simulink model "testTorchTCP"  (R2023b)
settings: Solver=FixedStepAuto  StartTime=0.0  StopTime=10.0  FixedStep=1  RelTol=1e-3
undefined symbols (not defined in the file or in its folder): inputDataStruct
libraries: instrumentlib x2
settings Model: Creator=pietr  LastModifiedBy=peterc

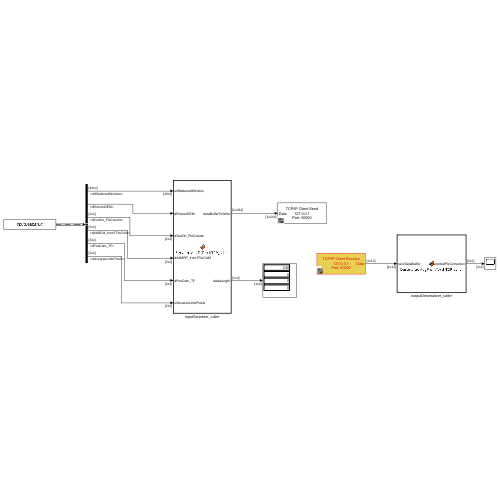
[thumbnail: Simulink's stored preview of the top-level diagram]
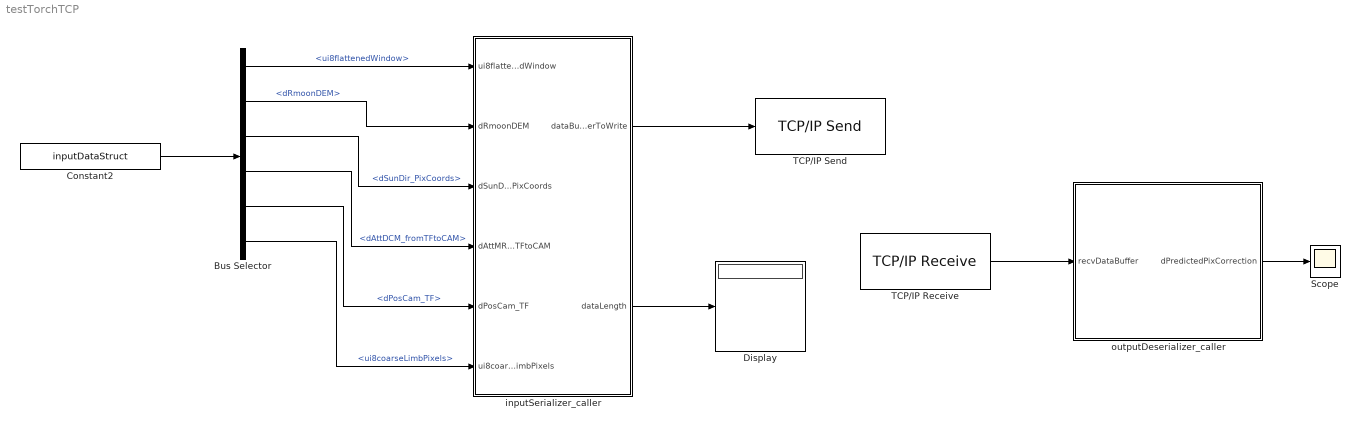
== system testTorchTCP ==
  Bus Selector : BusSelector  OutputSignals=ui8flattenedWindow,dRmoonDEM,dSunDir_PixCoords,dAttDCM_fromTFtoCAM,dPosCam_TF,ui8coarseLimbPixels
  Constant2 : Constant  Value=inputDataStruct  OutDataTypeStr=Bus: InputTorchModelBus  SampleTime=Inf
  Display : Display
  Scope : Scope
  TCP/IP Receive : instrumentlib/TCP//IP Receive  Host=127.0.0.1  Port=50000  DataSize=[1,12]  DataType=uint8  ASCIIFormatting=%f  Terminator=LF  CustomTerminator=10  ByteOrder=big-endian  EnableBlockingMode=on  Timeout=20  SampleTime=-1  SimulateUsing=Interpreted execution
  TCP/IP Send : instrumentlib/TCP//IP Send  Host=127.0.0.1  Port=50000  ByteOrder=little-endian  EnableBlockingMode=on  Timeout=10  TransferDelay=on  SimulateUsing=Interpreted execution
  inputSerializer_caller : MATLAB Function  TreatAsAtomicUnit=on
  outputDeserializer_caller : MATLAB Function  TreatAsAtomicUnit=on
  wires:
  outputDeserializer_caller/1(dPredictedPixCorrection) -> Scope/1
  inputSerializer_caller/1(dataBufferToWrite) -> TCP/IP Send/1
  inputSerializer_caller/2(dataLength) -> Display/1
  TCP/IP Receive/1 -> outputDeserializer_caller/1(recvDataBuffer)
  Constant2/1 -> Bus Selector/1
  Bus Selector/1 -> inputSerializer_caller/1(ui8flattenedWindow)  "<ui8flattenedWindow>"
  Bus Selector/2 -> inputSerializer_caller/2(dRmoonDEM)  "<dRmoonDEM>"
  Bus Selector/3 -> inputSerializer_caller/3(dSunDir_PixCoords)  "<dSunDir_PixCoords>"
  Bus Selector/4 -> inputSerializer_caller/4(dAttMRP_fromTFtoCAM)  "<dAttDCM_fromTFtoCAM>"
  Bus Selector/5 -> inputSerializer_caller/5(dPosCam_TF)  "<dPosCam_TF>"
  Bus Selector/6 -> inputSerializer_caller/6(ui8coarseLimbPixels)  "<ui8coarseLimbPixels>"

== matlab function testTorchTCP/outputDeserializer_caller ==
  data: recvDataBuffer input; dPredictedPixCorrection output
function dPredictedPixCorrection = DeserializeMsgFromTorchTCP_caller(recvDataBuffer)

recvBytes   = typecast(recvDataBuffer(1:4), 'int32');
recvDataBuffer_withoutLength = recvDataBuffer(5:end);

dPredictedPixCorrection = zeros(2,1,'double');

[dPredictedPixCorrection(:)] = DeserializeMsgFromTorchTCP(recvBytes, recvDataBuffer_withoutLength);

== matlab function testTorchTCP/inputSerializer_caller ==
  data: dataBufferToWrite output; dataLength output; ui8flattenedWindow input; dRmoonDEM input; dSunDir_PixCoords input; dAttMRP_fromTFtoCAM input; dPosCam_TF input; ui8coarseLimbPixels input
function [dataBufferToWrite, dataLength] = SerializeMsgToTorchTCP_caller(ui8flattenedWindow, ...
    dRmoonDEM, ...
    dSunDir_PixCoords, ...
    dAttMRP_fromTFtoCAM, ...
    dPosCam_TF, ...
    ui8coarseLimbPixels)

dataBufferToWrite = zeros(1,244,'uint8');
dataLength  = zeros(1,4,'uint8');

[dataLength(:), dataBufferToWrite(:)] = SerializeMsgToTorchTCP(ui8flattenedWindow, ...
    dRmoonDEM, ...
    dSunDir_PixCoords, ...
    dAttMRP_fromTFtoCAM, ...
    dPosCam_TF, ...
    ui8coarseLimbPixels);
